simulink model "System_without_Observer"  (Simulink 8.2)
settings: Solver=ode4  SolverMode=SingleTasking  StartTime=0.0  StopTime=Tend  FixedStep=0.0001  RelTol=1e-3
values from neighbouring files (symbols this model uses):
  Ax = [   0      Km/J         0 ... (first row only)    [Synthesis_SS_Controller.m]
  Bu = [0; 0; Kpc/Tpc]    [Synthesis_SS_Controller.m]
  C2 = eye(3,3)    [Synthesis_SS_Controller.m]
  Cx = [Kvs 0 0]    [Synthesis_SS_Controller.m]
  D2 = [0; 0; 0]    [Synthesis_SS_Controller.m]
  g = 1    [Synthesis_SS_Controller.m]
  Kg = 1/Ksys    [Synthesis_SS_Controller.m]
  KK = place(Ax, Bu, P)    [Synthesis_SS_Controller.m]
  X0 = [0; 0; 0]    [Synthesis_SS_Controller.m]
settings Model: Creator=RIS  LastModifiedBy=RIS
settings DataIOCC: SignalLoggingSaveFormat=Dataset
settings OptimizationCC: ExpressionDepthLimit=128
settings DebuggingCC: FcnCallInpInsideContextMsg=EnableAllAsError  StateNameClashWarn=none
settings GRTTargetCC: CombineOutputUpdateFcns=on  GRTInterface=off

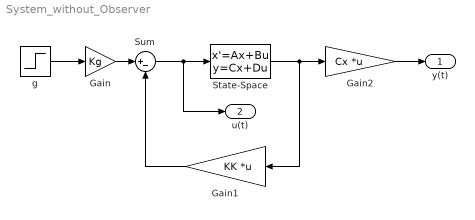
== system System_without_Observer ==
  Gain : Gain  Gain=Kg
  Gain1 : Gain  Gain=KK  Multiplication=Matrix(K*u) (u vector)
  Gain2 : Gain  Gain=Cx  Multiplication=Matrix(K*u) (u vector)
  State-Space : StateSpace  A=Ax  B=Bu  C=C2  D=D2  X0=X0
  Sum : Sum  Inputs=|+-
  g : Step  Time=0  After=g  SampleTime=0
  y(t) : Outport
  u(t) : Outport  Port=2
  wires:
  Sum/1 -> u(t)/1, State-Space/1
  Gain/1 -> Sum/1
  g/1 -> Gain/1
  State-Space/1 -> Gain1/1, Gain2/1
  Gain1/1 -> Sum/2
  Gain2/1 -> y(t)/1
